simulink model "MSFartoystyring_2_4"  (R2017b)
settings: Solver=ode45  StartTime=tstart  StopTime=tstop  RelTol=1e-3  EnableMultiTasking=on
values from neighbouring files (symbols this model uses):
  c = 1    [run_task_2_4.m]
  e_u_limit = 3    [run_task_2_4.m]
  Ki_u = 0.08    [run_task_2_4.m]
  Kp_los = 1/Delta    (= 0.00131233595801)    [run_task_2_4.m]
  Kp_u = 80    [run_task_2_4.m]
  p0 = [1500 500]'    [run_task_2_4.m]
  psi0 = 50*deg2rad    (= 0.872664625997)    [run_task_2_4.m]
  r0 = 0    [run_task_2_4.m]
  R_change_wp = 500    [run_task_2_4.m]
  r_d = 0*deg2rad    (= 0)    [run_task_2_4.m]
  R_vel = 300    [run_task_2_4.m]
  tsamp = 10    [run_task_2_4.m]
  v0 = [6.63 0]'    [run_task_2_4.m]
  wp = [p0 wp.WP]    [run_task_2_4.m]
undefined symbols (not defined in the file or in its folder): Kd_psi, Ki_psi, Ki_r, Kp_psi, Kp_r, msfartoystyring
settings Model: ExtModeAutoUpdateStatusClock=off  Creator=christh  LastModifiedBy=Alexandra
settings DataIOCC: LimitDataPoints=on  SaveFormat=Array  SignalLoggingSaveFormat=ModelDataLogs
settings OptimizationCC: ExpressionDepthLimit=2147483647  InitFltsAndDblsToZero=on  LifeSpan=inf
settings DebuggingCC: UnderspecifiedInitializationDetection=Classic  MergeDetectMultiDrivingBlocksExec=none  SolverPrmCheckMsg=warning  FcnCallInpInsideContextMsg=warning  StateNameClashWarn=warning  SFUnexpectedBacktrackingDiag=warning  SFNoUnconditionalDefaultTransitionDiag=warning  SFExecutionAtInitializationDiag=none
settings HardwareCC: ProdBitPerPointer=32  ProdBitPerSizeT=32  ProdBitPerPtrDiffT=32  ProdLargestAtomicFloat=None  ProdIntDivRoundTo=Undefined  ProdEndianess=Unspecified  ProdWordSize=32  ProdHWDeviceType=32-bit Generic
settings ModelReferenceCC: PropagateSignalLabelsOutOfModel=off
settings CodeAppCC: StateflowObjectComments=on
settings GRTTargetCC: TargetLangStandard=C89/C90 (ANSI)  GeneratePreprocessorConditionals=Disable all  CombineOutputUpdateFcns=off  GRTInterface=on
settings ConfigComp: CovMetricSettings=dw  CovHtmlReporting=on  CovSaveCumulativeToWorkspaceVar=on  CovSaveSingleToWorkspaceVar=on  CovExternalEMLEnable=off

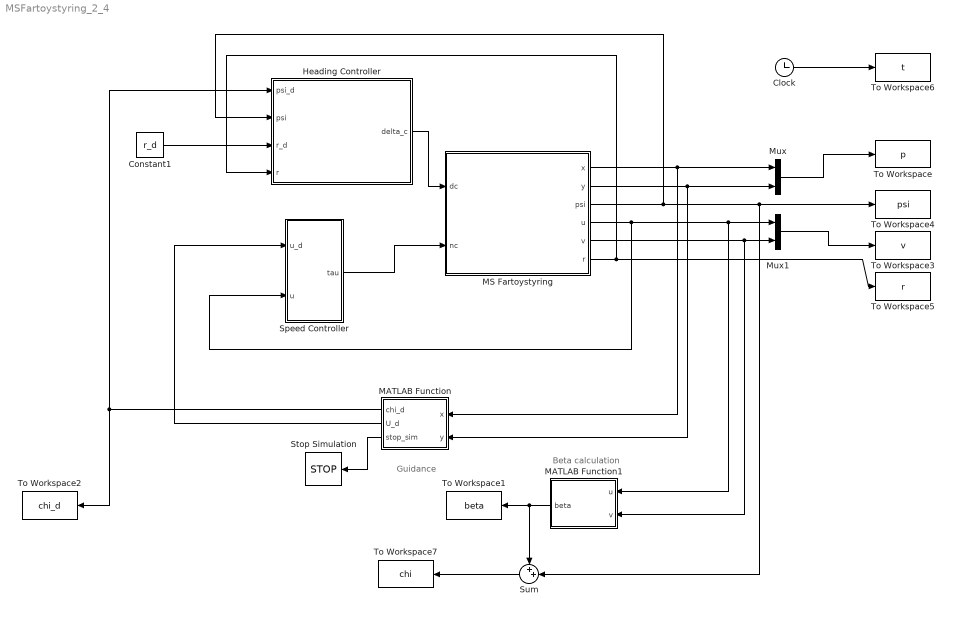
== system MSFartoystyring_2_4 ==
  note: Beta calculation
  note: Guidance
  Clock : Clock
  Constant1 : Constant  Value=r_d
  Heading Controller : Subsystem
  MATLAB Function : MATLAB Function  TreatAsAtomicUnit=on
  MATLAB Function1 : MATLAB Function  TreatAsAtomicUnit=on
  MS Fartoystyring : Subsystem  mask(MS Fartoystyring for Assignment 3 G&C){x0=p0(1), y0=p0(2), u0=v0(1), v0=v0(2), psi0=psi0, r0=r0, c=c}
      mask prompts: x0 "x(t0) (m)"; y0 "y(t0) (m)"; u0 "u(t0) (m/s)"; v0 "v(t0) (m/s)"; psi0 "psi(t0) (rad)"; r0 "r(t0) (rad/s)"; c "current (0 or 1)"
      mask help:
      | Block corresponding to Figure 1 in the assignment text. Gives the response of the ship.
      |
      | The design speed of MS Fartoystyring is u=8.23 m/s.
      |
      | Input:
      | dc: commanded rudder (rad), dmax=25*pi/180
      | nc: commanded shaft speed (rad/s), nmax=85*2*pi/60
      |
      | Output:
      | x: north pos (m)
      | y: east pos (m)
      | u: surge (m/s)
      | v: sway (m/s)
      | psi: heading (rad)
      | r: yaw (rad/s)
      mask Help: Comments, bugs and help requests can be directed to the TA. Email on course website.
  Mux : Mux  Inputs=2
  Mux1 : Mux  Inputs=2
  Speed Controller : Subsystem
  Stop Simulation : Stop
  Sum : Sum  Inputs=++|
  To Workspace : ToWorkspace  VariableName=p  SampleTime=tsamp
  To Workspace1 : ToWorkspace  VariableName=beta  SampleTime=tsamp
  To Workspace2 : ToWorkspace  VariableName=chi_d  SampleTime=tsamp
  To Workspace3 : ToWorkspace  VariableName=v  SampleTime=tsamp
  To Workspace4 : ToWorkspace  VariableName=psi  SampleTime=tsamp
  To Workspace5 : ToWorkspace  VariableName=r  SampleTime=tsamp
  To Workspace6 : ToWorkspace  VariableName=t  SampleTime=tsamp
  To Workspace7 : ToWorkspace  VariableName=chi  SampleTime=tsamp
  wires:
  Clock/1 -> To Workspace6/1
  MS Fartoystyring/1(x) -> Mux/1, MATLAB Function/1(x)
  MS Fartoystyring/2(y) -> MATLAB Function/2(y), Mux/2
  MS Fartoystyring/4(u) -> Speed Controller/2(u), MATLAB Function1/1(u), Mux1/1
  MS Fartoystyring/5(v) -> MATLAB Function1/2(v), Mux1/2
  Mux/1 -> To Workspace/1
  Mux1/1 -> To Workspace3/1
  Constant1/1 -> Heading Controller/3(r_d)
  MS Fartoystyring/6(r) -> Heading Controller/4(r), To Workspace5/1
  MATLAB Function/1(chi_d) -> To Workspace2/1, Heading Controller/1("psi_d ")
  Heading Controller/1(delta_c) -> MS Fartoystyring/1(dc)
  MATLAB Function/2(U_d) -> Speed Controller/1(u_d)
  Speed Controller/1(tau) -> MS Fartoystyring/2(nc)
  MATLAB Function/3(stop_sim) -> Stop Simulation/1
  MATLAB Function1/1(beta) -> Sum/1, To Workspace1/1
  MS Fartoystyring/3(psi) -> Heading Controller/2(psi), Sum/2, To Workspace4/1
  Sum/1 -> To Workspace7/1

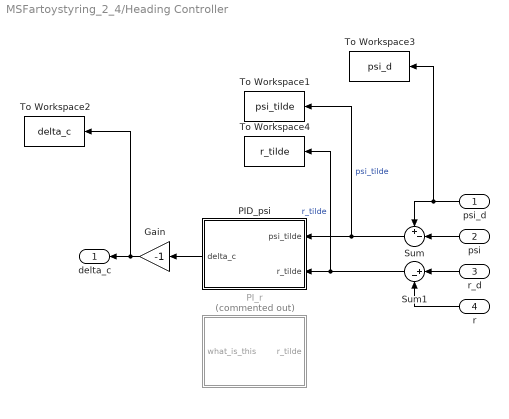
== system MSFartoystyring_2_4/Heading Controller ==
  "psi_d " : Inport
  psi : Inport  Port=2
  r_d : Inport  Port=3
  r : Inport  Port=4
  Gain : Gain  Gain=-1
  PID_psi : Subsystem
  PI_r : Subsystem  Commented=on
  Sum : Sum  Inputs=+-|
  Sum1 : Sum  Inputs=|+-
  To Workspace1 : ToWorkspace  VariableName=psi_tilde  SampleTime=tsamp
  To Workspace2 : ToWorkspace  VariableName=delta_c  SampleTime=tsamp
  To Workspace3 : ToWorkspace  VariableName=psi_d  SampleTime=tsamp
  To Workspace4 : ToWorkspace  VariableName=r_tilde  SampleTime=tsamp
  delta_c : Outport
  wires:
  psi/1 -> Sum/2
  "psi_d "/1 -> To Workspace3/1, Sum/1
  Sum1/1 -> To Workspace4/1, PID_psi/2(r_tilde)  "r_tilde"
  r_d/1 -> Sum1/1
  Sum/1 -> To Workspace1/1, PID_psi/1(psi_tilde)  "psi_tilde"
  r/1 -> Sum1/2
  Gain/1 -> To Workspace2/1, delta_c/1
  PID_psi/1(delta_c) -> Gain/1

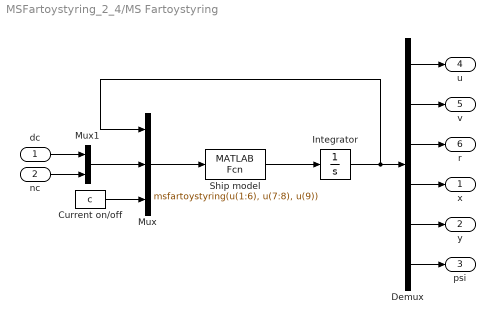
== system MSFartoystyring_2_4/MS Fartoystyring ==
  dc : Inport
  nc : Inport  Port=2
  Current on/off : Constant  Value=c
  Demux : Demux  Outputs=6
  Integrator : Integrator  InitialCondition=[u0 v0 r0 x0 y0 psi0]'
  Mux : Mux  Inputs=3
  Mux1 : Mux  Inputs=2
  Ship model : MATLABFcn  MATLABFcn=msfartoystyring(u(1:6), u(7:8), u(9))  OutputDimensions=6
  x : Outport
  y : Outport  Port=2
  psi : Outport  Port=3
  u : Outport  Port=4
  v : Outport  Port=5
  r : Outport  Port=6
  wires:
  Integrator/1 -> Mux/1, Demux/1
  Mux1/1 -> Mux/2
  dc/1 -> Mux1/1
  nc/1 -> Mux1/2
  Demux/1 -> u/1
  Demux/2 -> v/1
  Demux/3 -> r/1
  Demux/4 -> x/1
  Demux/5 -> y/1
  Demux/6 -> psi/1
  Current on/off/1 -> Mux/3
  Ship model/1 -> Integrator/1
  Mux/1 -> Ship model/1

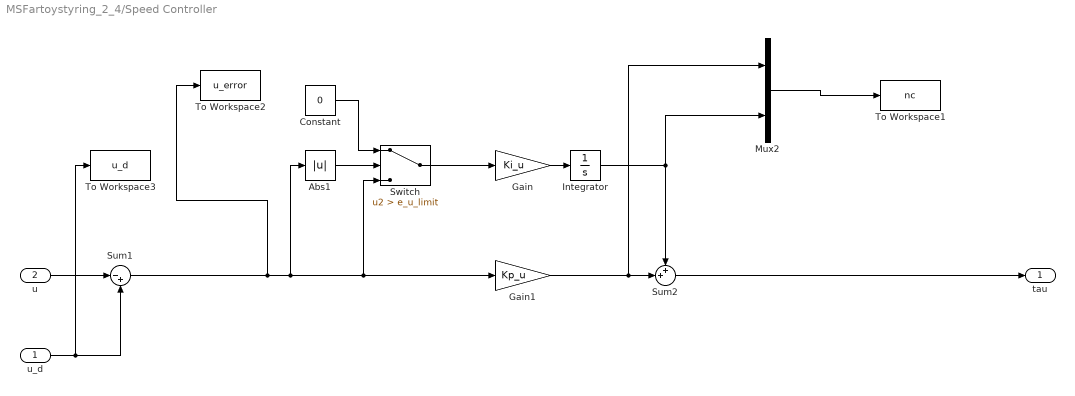
== system MSFartoystyring_2_4/Speed Controller ==
  u_d : Inport
  u : Inport  Port=2
  Abs1 : Abs
  Constant : Constant  Value=0
  Gain : Gain  Gain=Ki_u
  Gain1 : Gain  Gain=Kp_u
  Integrator : Integrator
  Mux2 : Mux  Inputs=2
  Sum1 : Sum  Inputs=|-+
  Sum2 : Sum  Inputs=++|
  Switch : Switch  Criteria=u2 > Threshold  Threshold=e_u_limit
  To Workspace1 : ToWorkspace  VariableName=nc  SampleTime=tsamp
  To Workspace2 : ToWorkspace  VariableName=u_error  SaveFormat=Structure With Time  SampleTime=tsamp
  To Workspace3 : ToWorkspace  VariableName=u_d  SaveFormat=Structure With Time  SampleTime=tsamp
  tau : Outport
  wires:
  Gain/1 -> Integrator/1
  Mux2/1 -> To Workspace1/1
  Abs1/1 -> Switch/2
  Constant/1 -> Switch/1
  Switch/1 -> Gain/1
  Gain1/1 -> Mux2/1, Sum2/2
  Integrator/1 -> Mux2/2, Sum2/1
  u/1 -> Sum1/1
  u_d/1 -> To Workspace3/1, Sum1/2
  Sum2/1 -> tau/1
  Sum1/1 -> To Workspace2/1, Switch/3, Gain1/1, Abs1/1

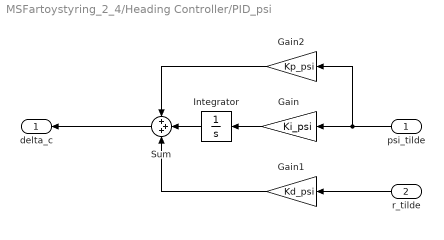
== system MSFartoystyring_2_4/Heading Controller/PID_psi ==
  psi_tilde : Inport
  r_tilde : Inport  Port=2
  Gain : Gain  Gain=Ki_psi
  Gain1 : Gain  Gain=Kd_psi
  Gain2 : Gain  Gain=Kp_psi
  Integrator : Integrator
  Sum : Sum  Inputs=+++
  delta_c : Outport
  wires:
  Gain2/1 -> Sum/1
  r_tilde/1 -> Gain1/1
  Gain1/1 -> Sum/3
  psi_tilde/1 -> Gain2/1, Gain/1
  Sum/1 -> delta_c/1
  Gain/1 -> Integrator/1
  Integrator/1 -> Sum/2

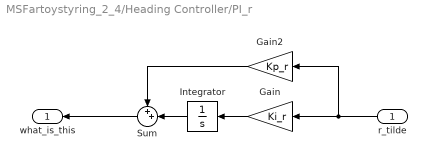
== system MSFartoystyring_2_4/Heading Controller/PI_r ==
  r_tilde : Inport
  Gain : Gain  Gain=Ki_r
  Gain2 : Gain  Gain=Kp_r
  Integrator : Integrator
  Sum : Sum  Inputs=++|
  what_is_this : Outport
  wires:
  Gain2/1 -> Sum/1
  r_tilde/1 -> Gain2/1, Gain/1
  Sum/1 -> what_is_this/1
  Gain/1 -> Integrator/1
  Integrator/1 -> Sum/2

== matlab function MSFartoystyring_2_4/MATLAB Function1 ==
  data: u input; beta output; v input
function beta = fcn(u, v)

beta = asin(v/sqrt(v^2+u^2));

end

== matlab function MSFartoystyring_2_4/MATLAB Function ==
  settings: updateMethod=DISCRETE  sampleTime=1
  data: chi_d output; x input; y input; U_d output; Kp_los parameter; R_vel parameter; R_change_wp parameter; wp parameter; stop_sim output
function [chi_d, U_d, stop_sim] = fcn(x, y, Kp_los, R_vel, R_change_wp, wp)

persistent k;

stop_sim = 0;

if isempty(k)
    k = 2;
end
% Get current waypoints
p_wp1 = wp(:,k-1);
p_wp2 = wp(:,k);

% Check acceptance Radius for change to next wp
if sqrt((p_wp2 - [x y]')'*(p_wp2 - [x y]')) <= R_change_wp
    k = k + 1;  
    if k <= size(wp,2)
        p_wp1 = wp(:,k-1);
        p_wp2 = wp(:,k);
    else
        disp('Were done here')
        stop_sim = 1;
    end
end


% % Check acceptance Radius for change of speed
% if (p_wp2 - [x y]')'*(p_wp2 - [x y]') <= R_vel
%     U_d = 5;  %m/s
% else
%     U_d = 10; %m/s
% end

U_d = 5;   % m/s

% Calculate chi_d
alpha = atan2(p_wp2(2)-p_wp1(2), p_wp2(1) - p_wp1(1));
p_b = [x y]';

Rp = [cos(alpha) -sin(alpha);
      sin(alpha) cos(alpha) ];
epsilon = Rp'*(p_b - p_wp1);
chi_d = mod(alpha + atan(-Kp_los*epsilon(2)), 2*pi);


end
